simulink subsystem "IntegratedElectromagnet"  (R2025a)
settings: Solver=VariableStepAuto  StartTime=0.0  StopTime=10.0  RelTol=1e-3
model mask{l_airgap=1e-09}
  mask prompts: l_airgap "initial air gap (mm) ="
libraries: fl_lib x6
settings Model: Creator=Polarstern  LastModifiedBy=CelestialAurora

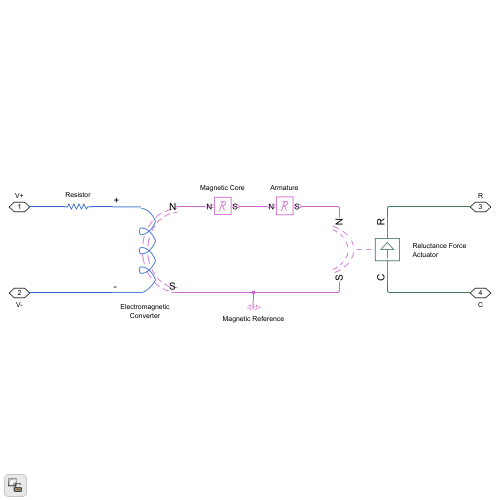
[thumbnail: Simulink's stored preview of the top-level diagram]
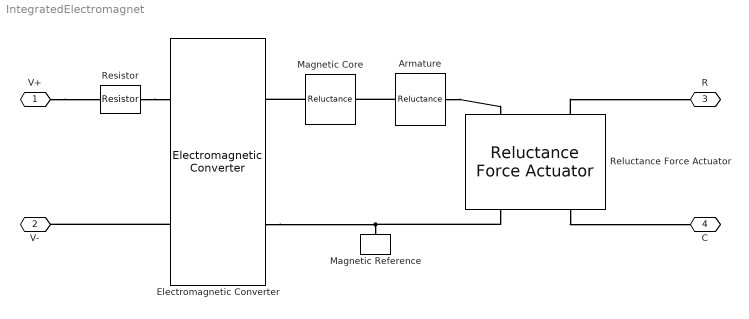
== system IntegratedElectromagnet ==
  Armature : fl_lib/Magnetic/Magnetic Elements/Reluctance  g=70 mm  CSA=0.0036 m^2  mur=5000  phi_specify=off  phi_priority=None  phi=0 Wb  phi_nominal_specify=off  phi_nominal_value=1  phi_nominal_unit=Wb  mmf_specify=off  mmf_priority=None  mmf=0 A  mmf_nominal_specify=off  mmf_nominal_value=1  mmf_nominal_unit=A
      settings: InternalSimscapePortConfiguration="{\"Bottom\":[],\"Left\":[{\"id\":\"N\",\"label\":\"N\",\"type\":\"foundation.magnetic.magnetic\"}],\"Right\":[{\"id\":\"S\",\"label\":\"S\",\"type\":\"foundation.magnetic.magnetic\"}],\"Top\":[]}"
  Electromagnetic Converter : fl_lib/Magnetic/Magnetic Elements/Electromagnetic Converter  Nw=100  i_specify=off  i_priority=None  i=0 A  i_nominal_specify=off  i_nominal_value=1  i_nominal_unit=A  v_specify=off  v_priority=None  v=0 V  v_nominal_specify=off  v_nominal_value=1  v_nominal_unit=V  mmf_specify=off  mmf_priority=None  mmf=0 A  mmf_nominal_specify=off  mmf_nominal_value=1  mmf_nominal_unit=A  phi_specify=on  phi_priority=Low  phi=0 Wb  phi_nominal_specify=off  phi_nominal_value=1  phi_nominal_unit=Wb
      settings: InternalSimscapePortConfiguration="{\"Bottom\":[],\"Left\":[{\"id\":\"p\",\"label\":\"+\",\"type\":\"foundation.electrical.electrical\"},{\"id\":\"n\",\"label\":\"-\",\"type\":\"foundation.electrical.electrical\"}],\"Right\":[{\"id\":\"N\",\"label\":\"N\",\"type\":\"foundation.magnetic.magnetic\"},{\"id\":\"S\",\"label\":\"S\",\"type\":\"foundation.magnetic.magnetic\"}],\"Top\":[]}"
  Magnetic Core : fl_lib/Magnetic/Magnetic Elements/Reluctance  g=170 mm  CSA=0.0072 m^2  mur=4000  phi_specify=off  phi_priority=None  phi=0 Wb  phi_nominal_specify=off  phi_nominal_value=1  phi_nominal_unit=Wb  mmf_specify=off  mmf_priority=None  mmf=0 A  mmf_nominal_specify=off  mmf_nominal_value=1  mmf_nominal_unit=A
      settings: InternalSimscapePortConfiguration="{\"Bottom\":[],\"Left\":[{\"id\":\"N\",\"label\":\"N\",\"type\":\"foundation.magnetic.magnetic\"}],\"Right\":[{\"id\":\"S\",\"label\":\"S\",\"type\":\"foundation.magnetic.magnetic\"}],\"Top\":[]}"
  Magnetic Reference : fl_lib/Magnetic/Magnetic Elements/Magnetic Reference
      settings: InternalSimscapePortConfiguration="{\"Bottom\":[],\"Left\":[{\"id\":\"M\",\"label\":\"\",\"type\":\"foundation.magnetic.magnetic\"}],\"Right\":[],\"Top\":[]}"
  Reluctance Force Actuator : fl_lib/Magnetic/Magnetic Elements/Reluctance Force Actuator  x0=l_airgap mm  xmin=1e-09 mm  CSA=0.0144 m^2  mur=1  K_contact=100000 N/m  D_contact=5000 N*s/m  mmf_specify=off  mmf_priority=None  mmf=0 A  mmf_nominal_specify=off  mmf_nominal_value=1  mmf_nominal_unit=A  phi_specify=off  phi_priority=None  phi=0 Wb  phi_nominal_specify=off  phi_nominal_value=1  phi_nominal_unit=Wb  f_specify=off  f_priority=None  f=0 N  f_nominal_specify=off  f_nominal_value=1  f_nominal_unit=N  u_specify=off  u_priority=None  u=0 m/s  u_nominal_specify=off  u_nominal_value=1  u_nominal_unit=m/s
      settings: InternalSimscapePortConfiguration="{\"Bottom\":[],\"Left\":[{\"id\":\"N\",\"label\":\"N\",\"type\":\"foundation.magnetic.magnetic\"},{\"id\":\"R\",\"label\":\"R\",\"type\":\"foundation.mechanical.translational.translational\"}],\"Right\":[{\"id\":\"S\",\"label\":\"S\",\"type\":\"foundation.magnetic.magnetic\"},{\"id\":\"C\",\"label\":\"C\",\"type\":\"foundation.mechanical.translational.translational\"}],\"Top\":[]}"
  Resistor : fl_lib/Electrical/Electrical Elements/Resistor  R=0.2 Ohm  i_specify=off  i_priority=None  i=0 A  i_nominal_specify=off  i_nominal_value=1  i_nominal_unit=A  v_specify=off  v_priority=None  v=0 V  v_nominal_specify=off  v_nominal_value=1  v_nominal_unit=V
  V+ : PMIOPort  Side=Left
  V- : PMIOPort  Port=2  Side=Left
  R : PMIOPort  Port=3  Side=Right
  C : PMIOPort  Port=4  Side=Right
  connections:
  Electromagnetic Converter/RConn2 -- Reluctance Force Actuator/RConn1 -- Magnetic Reference/LConn1
  Armature/RConn1 -- Reluctance Force Actuator/LConn1
  Magnetic Core/LConn1 -- Electromagnetic Converter/RConn1
  Resistor/RConn1 -- Electromagnetic Converter/LConn1
  V+/RConn1 -- Resistor/LConn1
  Armature/LConn1 -- Magnetic Core/RConn1
  Electromagnetic Converter/LConn2 -- V-/RConn1
  Reluctance Force Actuator/LConn2 -- R/RConn1
  Reluctance Force Actuator/RConn2 -- C/RConn1
